simulink model "motor_controller"  (R2023b)
settings: Solver=FixedStepAuto  StartTime=0.0  StopTime=10.0  RelTol=1e-3  EnableMultiTasking=on
model workspace (MAT data in the model file):
  FOC_Ts = Simulink.Parameter
  FOC_Ts.Value = 3.65714285714e-05
  FOC_Ts.DataType = 'auto'
  FOC_Ts.Complexity = 'real'
  FOC_Ts.Dimensions = [1 1]
  Outer_Ts = Simulink.Parameter
  Outer_Ts.Value = 0.001
  Outer_Ts.DataType = 'auto'
  Outer_Ts.Complexity = 'real'
  Outer_Ts.Dimensions = [1 1]
settings Model: DataDictionary=newBoard.sldd  Creator=mfussi  LastModifiedBy=mfussi
settings SolverCC: AutoInsertRateTranBlk=on  InsertRTBMode=Never (minimum delay)
settings GRTTargetCC: CodeInterfacePackaging=Reusable function  GenerateAllocFcn=on

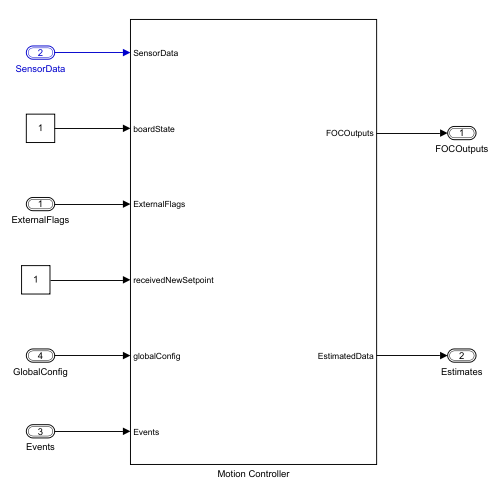
[thumbnail: Simulink's stored preview of the top-level diagram]
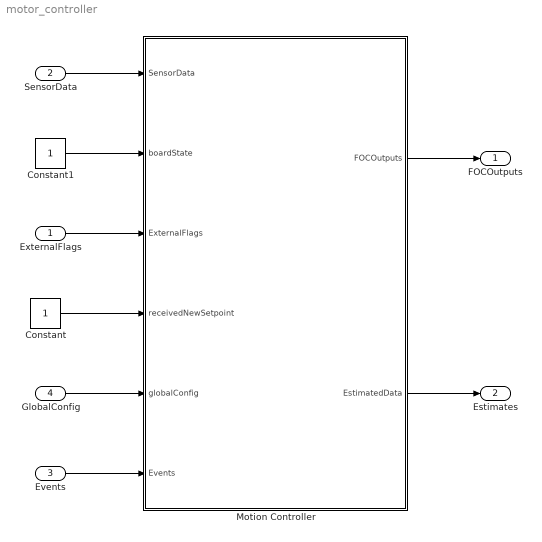
== system motor_controller ==
  ExternalFlags : Inport  OutDataTypeStr=Bus: ExternalFlags  BusOutputAsStruct=on
  SensorData : Inport  Port=2  OutDataTypeStr=Bus: SensorsData  SampleTime=FOC_Ts
  Events : Inport  Port=3  OutDataTypeStr=Bus: SupervisorReceivedEvents
  GlobalConfig : Inport  Port=4  OutDataTypeStr=Bus: GlobalConfiguration
  Constant : Constant  OutDataTypeStr=Inherit: Inherit via back propagation
  Constant1 : Constant
  Motion Controller : Subsystem
  FOCOutputs : Outport  OutDataTypeStr=Bus: FOCOutputs
  Estimates : Outport  Port=2  OutDataTypeStr=Bus: EstimatedData
  wires:
  SensorData/1 -> Motion Controller/1(SensorData)
  ExternalFlags/1 -> Motion Controller/3(ExternalFlags)
  Motion Controller/1(FOCOutputs) -> FOCOutputs/1
  Motion Controller/2(EstimatedData) -> Estimates/1
  Events/1 -> Motion Controller/6(Events)
  GlobalConfig/1 -> Motion Controller/5(globalConfig)
  Constant/1 -> Motion Controller/4(receivedNewSetpoint)
  Constant1/1 -> Motion Controller/2(boardState)

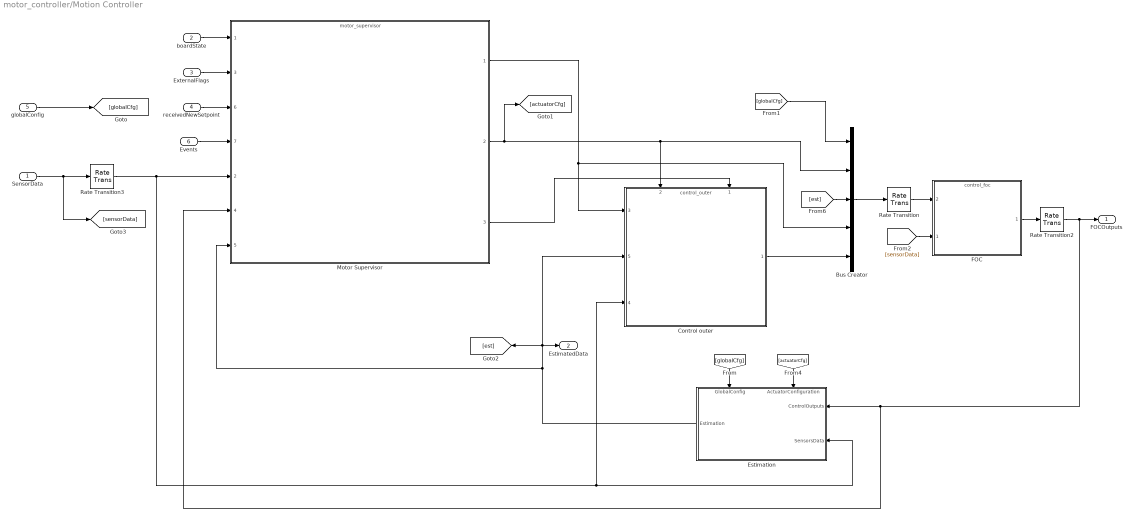
== system motor_controller/Motion Controller ==
  SensorData : Inport
  boardState : Inport  Port=2
  ExternalFlags : Inport  Port=3  OutDataTypeStr=Bus: ExternalFlags
  receivedNewSetpoint : Inport  Port=4
  globalConfig : Inport  Port=5
  Events : Inport  Port=6
  Bus Creator : BusCreator  Inputs=5  OutDataTypeStr=Bus: FOCSlowInputs  NonVirtualBus=on
      settings: InheritFromInputs=off
  Control outer : ModelReference  ModelNameDialog=control_outer.slx  SimulationMode=Normal  ModelReferenceVersion=6.7
      settings: PortSchema="{\"entries\":[{\"content\":{\"sides\":[{\"content\":{\"connectorIds\":[\"In3\",\"In5\",\"In4\"]},\"type\":\"ConnectorPlacement.EquallySpacedRectSide\",\"uuid\":\"5f0855f7-78ef-4761-b7b2-78e76d92fc4b\"},{\"content\":{\"connectorIds\":[\"Out1\"],\"side\":\"RIGHT\"},\"type\":\"ConnectorPlacement.EquallySpacedRectSide\",\"uuid\":\"ce4374cd-607c-4e0b-a8af-eb2e0e17051d\"},{\"content\":{\"connectorIds\":[\"In2\",\"In1\"],\"side\":\"TOP\"},\"type\":\"ConnectorPlacement.EquallySpacedRectSide\",\"uuid\":\"cef85d5e-e838-4f2a-8e72-80e83911c8d3\"},{\"content\":{\"side\":\"BOTTOM\"},\"type\":\"ConnectorPlacement.EquallySpacedRectSide\",\"uuid\":\"20390ec2-cce8-49cd-a78c-2a21c95dd133\"}]},\"type\":\"ConnectorPlacement.EquallySpacedConnector\",\"uuid\":\"234d6756-2ddf-48d1-9c55-249229e32550\"}],\"packageUris\":[\"http://schema.mathworks.com/mf0/Connector/R2020b\"],\"version\":\"1.0\"}"
  Estimation : Subsystem
      settings: PortSchema="{\"entries\":[{\"content\":{\"sides\":[{\"content\":{\"connectorIds\":[\"In1\",\"In2\"]},\"type\":\"ConnectorPlacement.EquallySpacedRectSide\",\"uuid\":\"180161ac-a548-41ce-8c3c-eb56a4bef2d5\"},{\"content\":{\"connectorIds\":[\"Out1\"],\"side\":\"RIGHT\"},\"type\":\"ConnectorPlacement.EquallySpacedRectSide\",\"uuid\":\"575f78f7-b1ab-47de-b691-5cd56a7f6610\"},{\"content\":{\"connectorIds\":[\"In3\",\"In4\"],\"side\":\"TOP\"},\"type\":\"ConnectorPlacement.EquallySpacedRectSide\",\"uuid\":\"318d42c0-b394-4491-8c9f-4e87fecabdd0\"}]},\"type\":\"ConnectorPlacement.EquallySpacedConnector\",\"uuid\":\"011ca5b5-9cf7-4201-870b-fa9d742ceb9c\"}],\"packageUris\":[\"http://schema.mathworks.com/mf0/Connector/R2020b\"],\"version\":\"1.0\"}"
  FOC : ModelReference  ModelNameDialog=control_foc.slx  SimulationMode=Normal  ModelReferenceVersion=6.24
      settings: PortSchema="{\"entries\":[{\"content\":{\"sides\":[{\"content\":{\"connectorIds\":[\"In2\",\"In1\"]},\"type\":\"ConnectorPlacement.EquallySpacedRectSide\",\"uuid\":\"ec9b0579-6bb0-408f-b762-24bae065c0be\"},{\"content\":{\"connectorIds\":[\"Out1\"],\"side\":\"RIGHT\"},\"type\":\"ConnectorPlacement.EquallySpacedRectSide\",\"uuid\":\"789a251a-9471-447b-a745-e431230ffa28\"},{\"content\":{\"side\":\"TOP\"},\"type\":\"ConnectorPlacement.EquallySpacedRectSide\",\"uuid\":\"ab802960-2701-40d7-b9cc-aaf192319073\"}]},\"type\":\"ConnectorPlacement.EquallySpacedConnector\",\"uuid\":\"0be03e7e-50b5-4985-b724-515ca9a23110\"}],\"packageUris\":[\"http://schema.mathworks.com/mf0/Connector/R2020b\"],\"version\":\"1.0\"}"
  Motor Supervisor : ModelReference  ModelNameDialog=motor_supervisor.slx  SimulationMode=Normal  ModelReferenceVersion=1.173
      settings: PortSchema="{\"entries\":[{\"content\":{\"sides\":[{\"content\":{\"connectorIds\":[\"In1\",\"In3\",\"In6\",\"In7\",\"In2\",\"In4\",\"In5\"]},\"type\":\"ConnectorPlacement.EquallySpacedRectSide\",\"uuid\":\"cef8e8ad-9c58-41ab-a08a-9ae722e40085\"},{\"content\":{\"connectorIds\":[\"Out1\",\"Out2\",\"Out3\"],\"side\":\"RIGHT\"},\"type\":\"ConnectorPlacement.EquallySpacedRectSide\",\"uuid\":\"f0f6bf4d-d146-4c52-85d0-e4a1fe2e14c9\"},{\"content\":{\"side\":\"TOP\"},\"type\":\"ConnectorPlacement.EquallySpacedRectSide\",\"uuid\":\"118dcde8-f32d-4dec-aaf2-5a7aa823a04d\"}]},\"type\":\"ConnectorPlacement.EquallySpacedConnector\",\"uuid\":\"5370414b-b8cf-4747-9f7c-0256206e2ab5\"}],\"packageUris\":[\"http://schema.mathworks.com/mf0/Connector/R2020b\"],\"version\":\"1.0\"}"
  Rate Transition : RateTransition  Deterministic=off  OutPortSampleTime=FOC_Ts
  Rate Transition2 : RateTransition  Deterministic=off  OutPortSampleTime=Outer_Ts
  Rate Transition3 : RateTransition  Deterministic=off  OutPortSampleTime=Outer_Ts
  FOCOutputs : Outport  OutDataTypeStr=Bus: FOCOutputs
  EstimatedData : Outport  Port=2
  wires:
  [est] -> Bus Creator/3
  Motor Supervisor/3 -> Control outer/1
  Motor Supervisor/2 -> [actuatorCfg], Bus Creator/2, Control outer/2
  Control outer/1 -> Bus Creator/5
  [actuatorCfg] -> Estimation/3(ActuatorConfiguration)
  Bus Creator/1 -> Rate Transition/1
  Estimation/1(Estimation) -> [est], Control outer/5, EstimatedData/1, Motor Supervisor/5
  Rate Transition2/1 -> Motor Supervisor/4, Estimation/1(ControlOutputs), FOCOutputs/1
  Rate Transition/1 -> FOC/2
  Motor Supervisor/1 -> Control outer/3, Bus Creator/4
  [globalCfg] -> Estimation/4(GlobalConfig)
  globalConfig/1 -> [globalCfg]
  [globalCfg] -> Bus Creator/1
  FOC/1 -> Rate Transition2/1
  Rate Transition3/1 -> Motor Supervisor/2, Control outer/4, Estimation/2(SensorsData)
  SensorData/1 -> [sensorData], Rate Transition3/1
  [sensorData] -> FOC/1
  receivedNewSetpoint/1 -> Motor Supervisor/6
  ExternalFlags/1 -> Motor Supervisor/3
  boardState/1 -> Motor Supervisor/1
  Events/1 -> Motor Supervisor/7

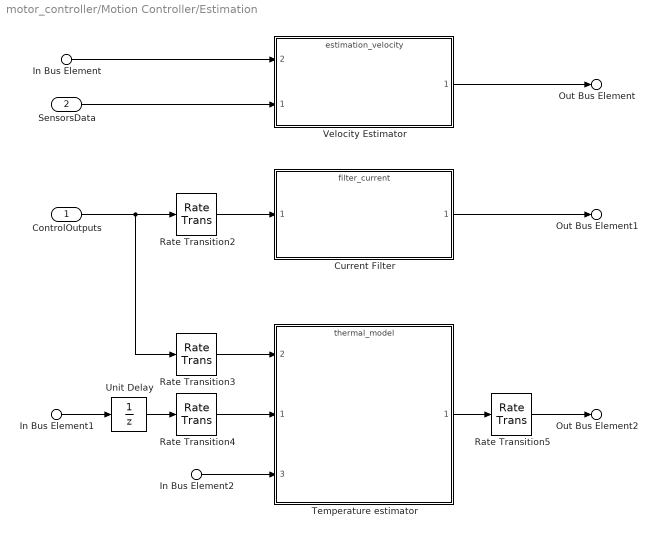
== system motor_controller/Motion Controller/Estimation ==
  ControlOutputs : Inport  OutDataTypeStr=Bus: FOCOutputs
  SensorsData : Inport  Port=2  OutDataTypeStr=Bus: SensorsData
  In Bus Element1 : Inport  Port=3  PortName=ActuatorConfiguration  Element=motor
  In Bus Element2 : Inport  Port=4  PortName=GlobalConfig  Element=estimation.environment_temperature
  In Bus Element : Inport  Port=4  PortName=GlobalConfig  Element=estimation.velocity_est_mode
  Current Filter : ModelReference  ModelNameDialog=filter_current.slx  SimulationMode=Normal  ModelReferenceVersion=6.2
  Rate Transition2 : RateTransition  Deterministic=off
  Rate Transition3 : RateTransition  Deterministic=off
  Rate Transition4 : RateTransition  Deterministic=off  OutPortSampleTime=1e-3
  Rate Transition5 : RateTransition  Deterministic=off
  Temperature estimator : ModelReference  ModelNameDialog=thermal_model.slx  SimulationMode=Normal  ModelReferenceVersion=6.10
      settings: PortSchema="{\"entries\":[{\"content\":{\"sides\":[{\"content\":{\"connectorIds\":[\"In2\",\"In1\",\"In3\"]},\"type\":\"ConnectorPlacement.EquallySpacedRectSide\",\"uuid\":\"78c786f4-5c3b-40e7-ad28-c0b961f14ec4\"},{\"content\":{\"connectorIds\":[\"Out1\"],\"side\":\"RIGHT\"},\"type\":\"ConnectorPlacement.EquallySpacedRectSide\",\"uuid\":\"b3487c62-68f2-43b6-a257-d51b1fb2e448\"},{\"content\":{\"side\":\"TOP\"},\"type\":\"ConnectorPlacement.EquallySpacedRectSide\",\"uuid\":\"5ce4df9e-b156-438c-989b-62dab6cef7f1\"}]},\"type\":\"ConnectorPlacement.EquallySpacedConnector\",\"uuid\":\"8f8c8caf-b0d2-4a2e-a596-6a6abf765763\"}],\"packageUris\":[\"http://schema.mathworks.com/mf0/Connector/R2020b\"],\"version\":\"1.0\"}"
  Unit Delay : UnitDelay  SampleTime=-1  HasFrameUpgradeWarning=on
  Velocity Estimator : ModelReference  ModelNameDialog=estimation_velocity.slx  SimulationMode=Normal  ModelReferenceVersion=6.7
      settings: PortSchema="{\"entries\":[{\"content\":{\"sides\":[{\"content\":{\"connectorIds\":[\"In2\",\"In1\"]},\"type\":\"ConnectorPlacement.EquallySpacedRectSide\",\"uuid\":\"ad3e0007-7e1a-45e3-9c4b-8557c15e59c9\"},{\"content\":{\"connectorIds\":[\"Out1\"],\"side\":\"RIGHT\"},\"type\":\"ConnectorPlacement.EquallySpacedRectSide\",\"uuid\":\"9939f2ed-714d-478a-b916-4c98246d3dad\"},{\"content\":{\"side\":\"TOP\"},\"type\":\"ConnectorPlacement.EquallySpacedRectSide\",\"uuid\":\"1f2bf02e-7550-4331-be09-78a4da3cd08c\"}]},\"type\":\"ConnectorPlacement.EquallySpacedConnector\",\"uuid\":\"c84d0359-7250-4a6f-b291-6b1b96be2690\"}],\"packageUris\":[\"http://schema.mathworks.com/mf0/Connector/R2020b\"],\"version\":\"1.0\"}"
  Out Bus Element : Outport  PortName=Estimation  Element=jointvelocities
  Out Bus Element1 : Outport  PortName=Estimation  Element=Iq_filtered
  Out Bus Element2 : Outport  PortName=Estimation  Element=motor_temperature
  wires:
  Temperature estimator/1 -> Rate Transition5/1
  Velocity Estimator/1 -> Out Bus Element/1
  Current Filter/1 -> Out Bus Element1/1
  In Bus Element1/1 -> Unit Delay/1
  SensorsData/1 -> Velocity Estimator/1
  ControlOutputs/1 -> Rate Transition2/1, Rate Transition3/1
  Rate Transition2/1 -> Current Filter/1
  Rate Transition3/1 -> Temperature estimator/2
  Rate Transition4/1 -> Temperature estimator/1
  Rate Transition5/1 -> Out Bus Element2/1
  Unit Delay/1 -> Rate Transition4/1
  In Bus Element/1 -> Velocity Estimator/2
  In Bus Element2/1 -> Temperature estimator/3
